simulink model "TBRe18_ECU_V7_AI"  (R2017b)
settings: Solver=FixedStepDiscrete  StartTime=0.0  StopTime=inf  FixedStep=0.0001  RelTol=1e-3
PostLoadFcn:
  | model_init();
libraries: simulink x16, simulink_extras x1
(part 1 of 4)
settings Model: SimulationMode=external  Creator=agf25  LastModifiedBy=kh469
settings DataIOCC: LimitDataPoints=on
settings OptimizationCC: DefaultParameterBehavior=Inlined  EfficientFloat2IntCast=on  LifeSpan=inf
settings DebuggingCC: AllowSymbolicDim=off  SFUnexpectedBacktrackingDiag=warning  SFNoUnconditionalDefaultTransitionDiag=warning  SFExecutionAtInitializationDiag=none
settings ModelReferenceCC: PropagateSignalLabelsOutOfModel=off
settings RTWCC: SystemTargetFile=nsi_mpc.tlc  MakeCommand=nsi_make  TemplateMakefile=nsi_mpc.tmf  Description=RTW Coder for MUXLAB4
settings CodeAppCC: StateflowObjectComments=on
settings STFCustomTargetCC: MATLABClassNameForMDSCustomization=Simulink.SoftwareTarget.TargetSpecificTriggerConfigurationBase  SystemTargetFile=nsi_mpc.tlc
settings ConfigComp: CovMetricSettings=dw  CovHtmlReporting=on  CovSaveCumulativeToWorkspaceVar=on  CovSaveSingleToWorkspaceVar=on  CovExternalEMLEnable=off
settings SimscapeCC: SimscapeNormalizeSystem=off
settings ConfigurationSet: Description=SimMechanics 2G

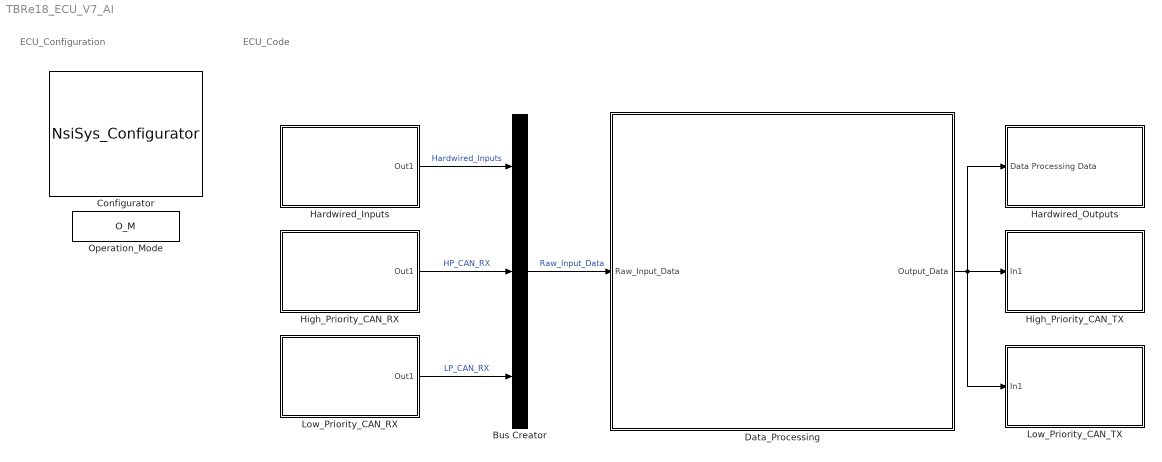
== system TBRe18_ECU_V7_AI ==
  note: ECU_Code
  note: ECU_Configuration
  Bus Creator : BusCreator  Inputs=3
  Configurator : S-Function  FunctionName=NsiSys_Configurator  Parameters=main,io,nbof_can,can,ccp,flash,nbof_lin,lin,tasks  SFunctionDeploymentMode=off  EnableBusSupport=off  mask(Configurator block){main=Config description;01/01/2011;0;0.000000, io=2.5;0;1;1;0;0;1;1;1, nbof_can=5, can=1;HIGH_SPEED;500Kbps;120 Ohm;C:\Users\TBRe-admin\Documents\MATLAB\TBRe18_DBC_190304.dbc;0;1;1Mbits;1;HIGH_SPEED;500Kbps;120 Ohm;C:\Users\TBRe-admin\Documents\MATLAB\TBRe18_DBC_190304.dbc;0;1;1Mbits;0;HIGH_SPEED;500Kbps;120 Ohm;C:\Users\l\Desktop\FYP\ECU\DBC\TBRe_DBC_V2.dbc;0;0;1Mbits;0;HIGH_SPEED;500Kbps;120 Ohm;D:\TOOLS\MUXLINK\R2011b\MUXlink\misc\j1939_adapt.dbc;0;1;1Mbits;0;HIGH_SPEED;1000Kbps;No;D:\TOOLS\MUXLINK\R2011b\MUXlink\misc\BASE_CAN_MUXLAB4.dbc;0;0;1Mbits, ccp=0;0x100;0x200;0;0;0x0;0x0;0;0x13, flash=Vehicle_STATE;No;Unsigned Byte;0;1;Operational_STATE;No;Unsigned Byte;0;1;Buzzer_time;No;Unsigned Byte;254;1;Buzzer_on;No;Boolean;1;1;reset_MEM;No;Boolean;0;1;TC_Slip_target;No;Unsigned Byte;5;1;TC_P_Gain;No;Unsigned Byte;1;1;TC_I_Gain;No;Unsigned Byte;1;1;TC_Offset;No;Signed Byte;0;1;DM_Mode;No;Unsigned Byte;0;1;DM_I_Gain;No;Unsigned Byte;1;1;IMD_MEM;No;Boolean;0;1;status_vehcle_LV;No;Boolean;0;1;status_vehcle_HV;No;Boolean;0;1;status_BMS;No;Boolean;0;1;status_IMD;No;Boolean;0;1;status_APPC;No;Boolean;0;1;status_APPS_BPPC;No;Boolean;0;1;status_RTD;No;Boolean;0;1;status_TC;No;Boolean;0;1;status_power_lim;No;Boolean;0;1;status_torque_derate;No;Boolean;0;1;status_tyre_radius;No;Unsigned Byte;22;1;power_limit;No;Unsigned Byte;30;1;torque_limit;No;Unsigned Byte;100;1, nbof_lin=2, lin=0;D:\TOOLS\MUXLINK\R2011b\MUXlink\misc\lindb.ldf;1;0.0;0.0;0.000;0.000;0.000000;0,0;0;D:\TOOLS\MUXLINK\R2011b\MUXlink\misc\lindb.ldf;1;0.0;0.0;0.000;0.000;0.000000;0,0, tasks=Data_Processing;[0.05];Hardwired_Inputs;[0.05];Hardwired_Outputs;[0.1];High_Priority_CAN_RX;[0.05];High_Priority_CAN_TX;[0.05];Low_Priority_CAN_RX;[0.05];Low_Priority_CAN_TX;[0.1]}
      mask prompts: nbof_can "nbof can"
      mask help: This block permits to set general parameters to use a MUXlink model
      mask init:
      | NsiSys_Configurator_InitializationFcn();
      settings: OpenFcn=NsiSys_Configurator_OpenFcn();
      mask Help:
      | eval('block=get_param(gcb, ''RTWdata'');')
      | web([docroot '\toolbox\MUXlink\html\blocks/' block.MUXlink_BlockType '.html'])
      mask Callback main: NsiSys_Configurator_ApplyFcn(1);
      mask Callback io: NsiSys_Configurator_ApplyFcn(2);
      mask Callback nbof_can: NsiSys_Configurator_ApplyFcn(3);
      mask Callback can: NsiSys_Configurator_ApplyFcn(4);
      mask Callback ccp: NsiSys_Configurator_ApplyFcn(5);
      mask Callback flash: NsiSys_Configurator_ApplyFcn(6);
      mask Callback nbof_lin: NsiSys_Configurator_ApplyFcn(7);
      mask Callback lin: NsiSys_Configurator_ApplyFcn(8);
      mask Callback tasks: NsiSys_Configurator_ApplyFcn(9);
      mask Display: image(imread('MUXLAB4.bmp'));text(0.5, 0.2, '', 'horizontalAlignment', 'center', 'verticalAlignment', 'base');
  Data_Processing : Subsystem  TreatAsAtomicUnit=on  SystemSampleTime=[0.05]  RTWFcnName=Data_Processing  RTWFileName=FileTaskFcn
      mask init:
      | NsiSys_SubSystemTask_InitializationFcn();
      settings: OpenFcn=NsiSys_SubSystemTask_OpenFcn();  RTWSystemCode=Nonreusable function  RTWFcnNameOpts=User specified  RTWFileNameOpts=Use function name
      mask Display: image(imread('nsi.bmp'));text(0.45, 0.9, 'task()');plot([0.05 0.05 0.05 0.05 0.05 0.05 0.05 0.05 0.05 0.05]);fprintf('Data_Processing\n/ 50.0ms / 10.0ms /\nEvent');
  Hardwired_Inputs : Subsystem  TreatAsAtomicUnit=on  SystemSampleTime=[0.05]  RTWFcnName=Hardwired_Inputs  RTWFileName=FileTaskFcn
      mask init:
      | NsiSys_SubSystemTask_InitializationFcn();
      settings: OpenFcn=NsiSys_SubSystemTask_OpenFcn();  RTWSystemCode=Nonreusable function  RTWFcnNameOpts=User specified  RTWFileNameOpts=Use function name
      mask Display: image(imread('nsi.bmp'));text(0.45, 0.9, 'task()');plot([0.05 0.05 0.05 0.05 0.05 0.05 0.05 0.05 0.05 0.05]);fprintf('Hardwired_Inputs\n/ 50.0ms / 0.0ms /\nEvent');
  Hardwired_Outputs : Subsystem  TreatAsAtomicUnit=on  SystemSampleTime=[0.1]  RTWFcnName=Hardwired_Outputs  RTWFileName=FileTaskFcn
      mask init:
      | NsiSys_SubSystemTask_InitializationFcn();
      settings: OpenFcn=NsiSys_SubSystemTask_OpenFcn();  RTWSystemCode=Nonreusable function  RTWFcnNameOpts=User specified  RTWFileNameOpts=Use function name
      mask Display: image(imread('nsi.bmp'));text(0.45, 0.9, 'task()');plot([0.05 0.05 0.05 0.05 0.05 0.05 0.05 0.05 0.05 0.05]);fprintf('Hardwired_Outputs\n/ 100.0ms / 0.0ms /\nEvent');
  High_Priority_CAN_RX : Subsystem  TreatAsAtomicUnit=on  SystemSampleTime=[0.05]  RTWFcnName=High_Priority_CAN_RX  RTWFileName=FileTaskFcn
      mask init:
      | NsiSys_SubSystemTask_InitializationFcn();
      settings: OpenFcn=NsiSys_SubSystemTask_OpenFcn();  RTWSystemCode=Nonreusable function  RTWFcnNameOpts=User specified  RTWFileNameOpts=Use function name
      mask Display: image(imread('nsi.bmp'));text(0.45, 0.9, 'task()');plot([0.05 0.05 0.05 0.05 0.05 0.05 0.05 0.05 0.05 0.05]);fprintf('High_Priority_CAN_RX\n/ 50.0ms / 0.0ms /\nEvent');
  High_Priority_CAN_TX : Subsystem  TreatAsAtomicUnit=on  SystemSampleTime=[0.05]  RTWFcnName=High_Priority_CAN_TX  RTWFileName=FileTaskFcn
      mask init:
      | NsiSys_SubSystemTask_InitializationFcn();
      settings: OpenFcn=NsiSys_SubSystemTask_OpenFcn();  RTWSystemCode=Nonreusable function  RTWFcnNameOpts=User specified  RTWFileNameOpts=Use function name
      mask Display: image(imread('nsi.bmp'));text(0.45, 0.9, 'task()');plot([0.05 0.05 0.05 0.05 0.05 0.05 0.05 0.05 0.05 0.05]);fprintf('High_Priority_CAN_TX\n/ 50.0ms / 20.0ms /\nEvent');
  Low_Priority_CAN_RX : Subsystem  TreatAsAtomicUnit=on  SystemSampleTime=[0.05]  RTWFcnName=Low_Priority_CAN_RX  RTWFileName=FileTaskFcn
      mask init:
      | NsiSys_SubSystemTask_InitializationFcn();
      settings: OpenFcn=NsiSys_SubSystemTask_OpenFcn();  RTWSystemCode=Nonreusable function  RTWFcnNameOpts=User specified  RTWFileNameOpts=Use function name
      mask Display: image(imread('nsi.bmp'));text(0.45, 0.9, 'task()');plot([0.05 0.05 0.05 0.05 0.05 0.05 0.05 0.05 0.05 0.05]);fprintf('Low_Priority_CAN_RX\n/ 50.0ms / 0.0ms /\nEvent');
  Low_Priority_CAN_TX : Subsystem  TreatAsAtomicUnit=on  SystemSampleTime=[0.1]  RTWFcnName=Low_Priority_CAN_TX  RTWFileName=FileTaskFcn
      mask init:
      | NsiSys_SubSystemTask_InitializationFcn();
      settings: OpenFcn=NsiSys_SubSystemTask_OpenFcn();  RTWSystemCode=Nonreusable function  RTWFcnNameOpts=User specified  RTWFileNameOpts=Use function name
      mask Display: image(imread('nsi.bmp'));text(0.45, 0.9, 'task()');plot([0.05 0.05 0.05 0.05 0.05 0.05 0.05 0.05 0.05 0.05]);fprintf('Low_Priority_CAN_TX\n/ 100.0ms / 0.0ms /\nEvent');
  Operation_Mode : DataStoreMemory  DataStoreName=O_M  ReadBeforeWriteMsg=warning  WriteAfterWriteMsg=warning  WriteAfterReadMsg=warning  ShowAdditionalParam=off
  wires:
  Low_Priority_CAN_RX/1(Out1) -> Bus Creator/3  "LP_CAN_RX"
  High_Priority_CAN_RX/1(Out1) -> Bus Creator/2  "HP_CAN_RX"
  Hardwired_Inputs/1(Out1) -> Bus Creator/1  "Hardwired_Inputs"
  Bus Creator/1 -> Data_Processing/1(Raw_Input_Data)  "Raw_Input_Data"
  Data_Processing/1(Output_Data) -> Low_Priority_CAN_TX/1(In1), High_Priority_CAN_TX/1(In1), Hardwired_Outputs/1(Data Processing Data)

== system TBRe18_ECU_V7_AI/Data_Processing ==
  note: Data_Processing
  Raw_Input_Data : Inport
  Diagnostics : Subsystem
  Init : Subsystem  mask(System Initialize){}
      mask help: Add code to a systems Initialize function
      settings: CopyFcn=cccopyfcn(gcb)  OpenFcn=ccopenfcn('System Initialize Function')
      mask Help: This block contains text fields to insert custom user code sections at the declaration, execution and exit sections of the systems initialize function.  By placing this block inside a subsytem, the custom user code will appear in that subsystems function.
      mask Display: disp('I()')
  Signal Conversion : SignalConversion  OverrideOpt=off
  Task : S-Function  FunctionName=NsiSys_TaskREF  Parameters=task_initialised,task_periodic, task_sampletime,task_name,task_event,task_offset  SFunctionDeploymentMode=off  EnableBusSupport=off  mask(task definition){task_initialised=on, task_periodic=on, task_sampletime=[0.05], task_offset=0.01, task_name=Data_Processing, task_event=on}
      mask prompts: task_initialised "task initialised"; task_periodic "Is Periodic"; task_sampletime "Task sample time"; task_offset "Task Offset"; task_name "Task name"; task_event "Is event"
      mask help:
      | Permit to provide all parameters associated to a MUXLINK task.
      | Task can be executed periodicaly and/or on event detection.
      | If task is periodic:
      | Task sample time specify the execution period in mS [0.001   6000]
      | Task Offset specify the offset applied to the execution period
      | Task Offset < Task sample time
      mask init:
      | NsiSys_TaskREF_InitializationFcn();
      settings: OpenFcn=NsiSys_Task_OpenFcn();
      mask Callback task_initialised: NsiSys_TaskREF_ApplyFcn(1);
      mask Callback task_periodic: NsiSys_TaskREF_ApplyFcn(2);
      mask Callback task_sampletime: NsiSys_TaskREF_ApplyFcn(3);
      mask Callback task_offset: NsiSys_TaskREF_ApplyFcn(6);
      mask Callback task_name: NsiSys_TaskREF_ApplyFcn(4);
      mask Callback task_event: NsiSys_TaskREF_ApplyFcn(5);
      mask Display: text(0.5, 0.8, 't()', 'horizontalAlignment', 'center', 'verticalAlignment', 'base');text(0.5, 0.2, '/ 50.0ms / 10.0ms /', 'horizontalAlignment', 'center', 'verticalAlignment', 'base');text(0.5, 0.4, 'Event', 'horizontalAlignment', 'center', 'verticalAlignment', 'base');
  Vehicle_Functionality : Subsystem
  Output_Data : Outport
  wires:
  Raw_Input_Data/1 -> Signal Conversion/1
  Diagnostics/1(Input_Data_Bus) -> Vehicle_Functionality/1(Input_Data)
  Signal Conversion/1 -> Diagnostics/1(Raw_Input_Data)
  Vehicle_Functionality/1(Output_Data_Bus) -> Output_Data/1

== system TBRe18_ECU_V7_AI/Hardwired_Inputs ==
  AnalogInput2 : S-Function  FunctionName=NsiIo_AnalogInput  Parameters=channel  SFunctionDeploymentMode=off  EnableBusSupport=off  mask(MUXlink I/O Analog Input){channel=7, RANGE=0 / 20 Volts}
      mask prompts: channel "Channel ?"; RANGE "Plage de mesure"
      mask help: This block interface the 8 Analog Inputs. Channels 1 to 4 are 0/10V, and the channels 5 to 8 are0/20V. Voltage input is read in mV
      mask init:
      | NsiIo_AnalogInput_InitializationFcn();
      settings: OpenFcn=NsiIo_AnalogInput_OpenFcn();
      mask Help:
      | eval('block=get_param(gcb, ''RTWdata'');')
      | web([docroot '\toolbox\MUXlink\html\blocks/' block.MUXlink_BlockType '.html'])
      mask Callback channel: NsiIo_AnalogInput_ApplyFcn();
      mask Callback RANGE: NsiIo_AnalogInput_ApplyFcn();
      mask Display: image(imread('nsi.bmp'));text(0.5, 0.2, 'AnalogInput_7\n\n0 / 20 Volts', 'horizontalAlignment', 'center', 'verticalAlignment', 'base');plot([0.05 0.05 0.05 0.05 0.05 0.05 0.05 0.05 0.05 0.05]);port_label('output', 1, 'D3');
  Bus Creator : BusCreator  Inputs=7
  Console : Subsystem
  DigitalInput1 : S-Function  FunctionName=NsiIo_DigitalInput  Parameters=channel,is_trigger,typeof_trigger,is_wakeup,wakeup_level  SFunctionDeploymentMode=off  EnableBusSupport=off  mask(MUXlink I/O Digital Input){channel=6, is_trigger=off, typeof_trigger=Either, is_wakeup=off, wakeup_level=Low level}
      mask prompts: channel "Channel ?"; is_trigger "Trigger ?"; typeof_trigger "Type of Trigger ?"; is_wakeup "Wake-up ?"; wakeup_level "Wake-up level ?"
      mask help: Read digital input from I/O channel.
      mask init:
      | NsiIo_DigitalInput_InitializationFcn();
      settings: OpenFcn=NsiIo_DigitalInput_OpenFcn();
      mask Help:
      | eval('block=get_param(gcb, ''RTWdata'');')
      | web([docroot '\toolbox\MUXlink\html\blocks/' block.MUXlink_BlockType '.html'])
      mask Callback channel: NsiIo_DigitalInput_ApplyFcn(1);
      mask Callback is_trigger: NsiIo_DigitalInput_ApplyFcn(2);
      mask TypeOptions typeof_trigger: Rising | Falling | Either
      mask Callback typeof_trigger: NsiIo_DigitalInput_ApplyFcn(3);
      mask Callback is_wakeup: NsiIo_DigitalInput_ApplyFcn(4);
      mask TypeOptions wakeup_level: Low level | High level
      mask Callback wakeup_level: NsiIo_DigitalInput_ApplyFcn(5);
      mask Display: image(imread('nsi.bmp'));text(0.5, 0.2, 'DigitalInput_6', 'horizontalAlignment', 'center', 'verticalAlignment', 'base');plot([0.05 0.05 0.05 0.05 0.05 0.05 0.05 0.05 0.05 0.05]);port_label('output', 1, 'Ground : B2');
  Ground : Ground
  Ground1 : Ground
  Init : Subsystem  mask(System Initialize){}
      mask help: Add code to a systems Initialize function
      settings: CopyFcn=cccopyfcn(gcb)  OpenFcn=ccopenfcn('System Initialize Function')
      mask Help: This block contains text fields to insert custom user code sections at the declaration, execution and exit sections of the systems initialize function.  By placing this block inside a subsytem, the custom user code will appear in that subsystems function.
      mask Display: disp('I()')
  Pedal_Box : Subsystem
  Task : S-Function  FunctionName=NsiSys_TaskREF  Parameters=task_initialised,task_periodic, task_sampletime,task_name,task_event,task_offset  SFunctionDeploymentMode=off  EnableBusSupport=off  mask(task definition){task_initialised=on, task_periodic=on, task_sampletime=[0.05], task_offset=0.0, task_name=Hardwired_Inputs, task_event=on}
      mask prompts: task_initialised "task initialised"; task_periodic "Is Periodic"; task_sampletime "Task sample time"; task_offset "Task Offset"; task_name "Task name"; task_event "Is event"
      mask help:
      | Permit to provide all parameters associated to a MUXLINK task.
      | Task can be executed periodicaly and/or on event detection.
      | If task is periodic:
      | Task sample time specify the execution period in mS [0.001   6000]
      | Task Offset specify the offset applied to the execution period
      | Task Offset < Task sample time
      mask init:
      | NsiSys_TaskREF_InitializationFcn();
      settings: OpenFcn=NsiSys_Task_OpenFcn();
      mask Callback task_initialised: NsiSys_TaskREF_ApplyFcn(1);
      mask Callback task_periodic: NsiSys_TaskREF_ApplyFcn(2);
      mask Callback task_sampletime: NsiSys_TaskREF_ApplyFcn(3);
      mask Callback task_offset: NsiSys_TaskREF_ApplyFcn(6);
      mask Callback task_name: NsiSys_TaskREF_ApplyFcn(4);
      mask Callback task_event: NsiSys_TaskREF_ApplyFcn(5);
      mask Display: text(0.5, 0.8, 't()', 'horizontalAlignment', 'center', 'verticalAlignment', 'base');text(0.5, 0.2, '/ 50.0ms / 0.0ms /', 'horizontalAlignment', 'center', 'verticalAlignment', 'base');text(0.5, 0.4, 'Event', 'horizontalAlignment', 'center', 'verticalAlignment', 'base');
  VBat : S-Function  FunctionName=NsiIo_Vbat  SFunctionDeploymentMode=off  EnableBusSupport=off  mask(MUXlink I/O VBat){}
      mask help: Battery Voltage
      mask init:
      | NsiIo_Vbat_InitializationFcn();
      settings: OpenFcn=NsiIo_Vbat_OpenFcn();
      mask Help:
      | eval('block=get_param(gcb, ''RTWdata'');')
      | web([docroot '\toolbox\MUXlink\html\blocks/' block.MUXlink_BlockType '.html'])
      mask Display: image(imread('nsi.bmp'));text(0.5, 0.2, 'I/O VBat', 'horizontalAlignment', 'center', 'verticalAlignment', 'base');plot([0.05 0.05 0.05 0.05 0.05 0.05 0.05 0.05 0.05 0.05]);port_label('output', 1, 'Voltage');
  Out1 : Outport
  wires:
  Pedal_Box/1(Out1) -> Bus Creator/1  "Pedal_Box_Data"
  Console/1(Out1) -> Bus Creator/2  "Console_Data"
  Bus Creator/1 -> Out1/1
  VBat/1 -> Bus Creator/3  "LV_Battery_Voltage"
  AnalogInput2/1 -> Bus Creator/7  "AMS_Ok"
  Ground/1 -> Bus Creator/4
  Ground1/1 -> Bus Creator/6
  DigitalInput1/1 -> Bus Creator/5  "RTD_Driverless"

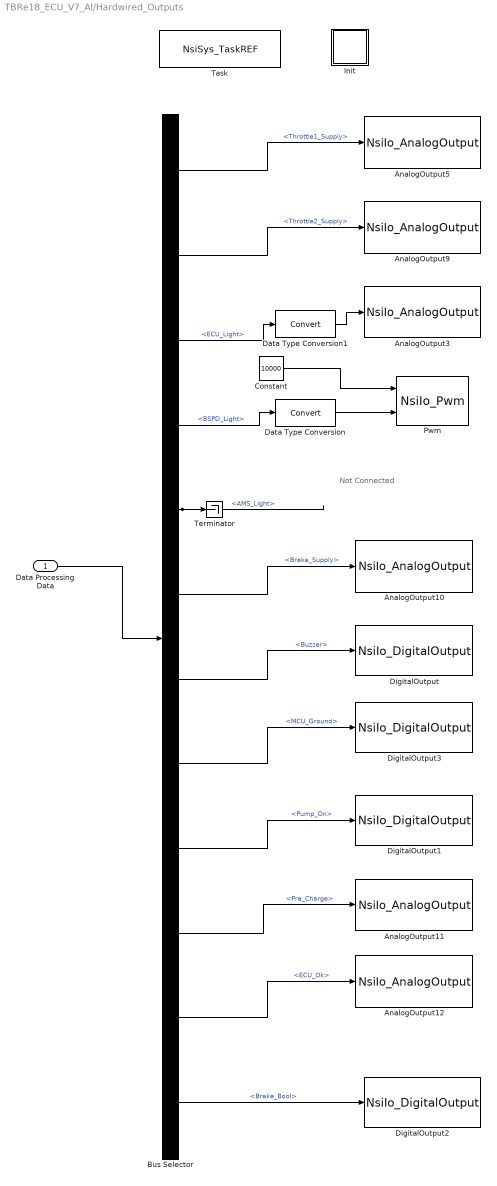
== system TBRe18_ECU_V7_AI/Hardwired_Outputs ==
  note: Not Connected
  Data Processing Data : Inport
  AnalogOutput10 : S-Function  Description=fsgqsdgqsgqsqs\nqdsjfhkqfkqsd  FunctionName=NsiIo_AnalogOutput  Parameters=Channel,Feedback  SFunctionDeploymentMode=off  EnableBusSupport=off  mask(MUXlink I/O Analog Output){Channel=5, Feedback=off, RANGE=0 / 20 Volts}
      mask prompts: Channel "Channel ?"; Feedback "Read Back Analog out"; RANGE "Voltage Range"
      mask help: This block interface the 8 Analog Outputs. Channels 1 to 4 are 0/10V, and the channels 5 to 8 are0/20V. Voltage input is set in mV
      mask init:
      | NsiIo_AnalogOutput_InitializationFcn();
      settings: OpenFcn=NsiIo_AnalogOutput_OpenFcn();
      mask Help:
      | eval('block=get_param(gcb, ''RTWdata'');')
      | web([docroot '\toolbox\MUXlink\html\blocks/' block.MUXlink_BlockType '.html'])
      mask Callback Channel: NsiIo_AnalogOutput_ApplyFcn(1);
      mask Display: image(imread('nsi.bmp'));text(0.5, 0.2, 'AnalogOutput_5\n\n0 / 20 Volts', 'horizontalAlignment', 'center', 'verticalAlignment', 'base');plot([0.05 0.05 0.05 0.05 0.05 0.05 0.05 0.05 0.05 0.05]);port_label('input', 1, 'F3');
  AnalogOutput11 : S-Function  Description=fsgqsdgqsgqsqs\nqdsjfhkqfkqsd  FunctionName=NsiIo_AnalogOutput  Parameters=Channel,Feedback  SFunctionDeploymentMode=off  EnableBusSupport=off  mask(MUXlink I/O Analog Output){Channel=7, Feedback=off, RANGE=0 / 20 Volts}
      mask prompts: Channel "Channel ?"; Feedback "Read Back Analog out"; RANGE "Voltage Range"
      mask help: This block interface the 8 Analog Outputs. Channels 1 to 4 are 0/10V, and the channels 5 to 8 are0/20V. Voltage input is set in mV
      mask init:
      | NsiIo_AnalogOutput_InitializationFcn();
      settings: OpenFcn=NsiIo_AnalogOutput_OpenFcn();
      mask Help:
      | eval('block=get_param(gcb, ''RTWdata'');')
      | web([docroot '\toolbox\MUXlink\html\blocks/' block.MUXlink_BlockType '.html'])
      mask Callback Channel: NsiIo_AnalogOutput_ApplyFcn(1);
      mask Display: image(imread('nsi.bmp'));text(0.5, 0.2, 'AnalogOutput_7\n\n0 / 20 Volts', 'horizontalAlignment', 'center', 'verticalAlignment', 'base');plot([0.05 0.05 0.05 0.05 0.05 0.05 0.05 0.05 0.05 0.05]);port_label('input', 1, 'A2');
  AnalogOutput12 : S-Function  Description=fsgqsdgqsgqsqs\nqdsjfhkqfkqsd  FunctionName=NsiIo_AnalogOutput  Parameters=Channel,Feedback  SFunctionDeploymentMode=off  EnableBusSupport=off  mask(MUXlink I/O Analog Output){Channel=2, Feedback=off, RANGE=0 / 20 Volts}
      mask prompts: Channel "Channel ?"; Feedback "Read Back Analog out"; RANGE "Voltage Range"
      mask help: This block interface the 8 Analog Outputs. Channels 1 to 4 are 0/10V, and the channels 5 to 8 are0/20V. Voltage input is set in mV
      mask init:
      | NsiIo_AnalogOutput_InitializationFcn();
      settings: OpenFcn=NsiIo_AnalogOutput_OpenFcn();
      mask Help:
      | eval('block=get_param(gcb, ''RTWdata'');')
      | web([docroot '\toolbox\MUXlink\html\blocks/' block.MUXlink_BlockType '.html'])
      mask Callback Channel: NsiIo_AnalogOutput_ApplyFcn(1);
      mask Display: image(imread('nsi.bmp'));text(0.5, 0.2, 'AnalogOutput_2\n\n0 / 20 Volts', 'horizontalAlignment', 'center', 'verticalAlignment', 'base');plot([0.05 0.05 0.05 0.05 0.05 0.05 0.05 0.05 0.05 0.05]);port_label('input', 1, 'E4');
  AnalogOutput3 : S-Function  Description=fsgqsdgqsgqsqs\nqdsjfhkqfkqsd  FunctionName=NsiIo_AnalogOutput  Parameters=Channel,Feedback  SFunctionDeploymentMode=off  EnableBusSupport=off  mask(MUXlink I/O Analog Output){Channel=6, Feedback=off, RANGE=0 / 20 Volts}
      mask prompts: Channel "Channel ?"; Feedback "Read Back Analog out"; RANGE "Voltage Range"
      mask help: This block interface the 8 Analog Outputs. Channels 1 to 4 are 0/10V, and the channels 5 to 8 are0/20V. Voltage input is set in mV
      mask init:
      | NsiIo_AnalogOutput_InitializationFcn();
      settings: OpenFcn=NsiIo_AnalogOutput_OpenFcn();
      mask Help:
      | eval('block=get_param(gcb, ''RTWdata'');')
      | web([docroot '\toolbox\MUXlink\html\blocks/' block.MUXlink_BlockType '.html'])
      mask Callback Channel: NsiIo_AnalogOutput_ApplyFcn(1);
      mask Display: image(imread('nsi.bmp'));text(0.5, 0.2, 'AnalogOutput_6\n\n0 / 20 Volts', 'horizontalAlignment', 'center', 'verticalAlignment', 'base');plot([0.05 0.05 0.05 0.05 0.05 0.05 0.05 0.05 0.05 0.05]);port_label('input', 1, 'F4');
  AnalogOutput5 : S-Function  Description=fsgqsdgqsgqsqs\nqdsjfhkqfkqsd  FunctionName=NsiIo_AnalogOutput  Parameters=Channel,Feedback  SFunctionDeploymentMode=off  EnableBusSupport=off  mask(MUXlink I/O Analog Output){Channel=3, Feedback=off, RANGE=0 / 20 Volts}
      mask prompts: Channel "Channel ?"; Feedback "Read Back Analog out"; RANGE "Voltage Range"
      mask help: This block interface the 8 Analog Outputs. Channels 1 to 4 are 0/10V, and the channels 5 to 8 are0/20V. Voltage input is set in mV
      mask init:
      | NsiIo_AnalogOutput_InitializationFcn();
      settings: OpenFcn=NsiIo_AnalogOutput_OpenFcn();
      mask Help:
      | eval('block=get_param(gcb, ''RTWdata'');')
      | web([docroot '\toolbox\MUXlink\html\blocks/' block.MUXlink_BlockType '.html'])
      mask Callback Channel: NsiIo_AnalogOutput_ApplyFcn(1);
      mask Display: image(imread('nsi.bmp'));text(0.5, 0.2, 'AnalogOutput_3\n\n0 / 20 Volts', 'horizontalAlignment', 'center', 'verticalAlignment', 'base');plot([0.05 0.05 0.05 0.05 0.05 0.05 0.05 0.05 0.05 0.05]);port_label('input', 1, 'F1');
  AnalogOutput9 : S-Function  Description=fsgqsdgqsgqsqs\nqdsjfhkqfkqsd  FunctionName=NsiIo_AnalogOutput  Parameters=Channel,Feedback  SFunctionDeploymentMode=off  EnableBusSupport=off  mask(MUXlink I/O Analog Output){Channel=4, Feedback=off, RANGE=0 / 20 Volts}
      mask prompts: Channel "Channel ?"; Feedback "Read Back Analog out"; RANGE "Voltage Range"
      mask help: This block interface the 8 Analog Outputs. Channels 1 to 4 are 0/10V, and the channels 5 to 8 are0/20V. Voltage input is set in mV
      mask init:
      | NsiIo_AnalogOutput_InitializationFcn();
      settings: OpenFcn=NsiIo_AnalogOutput_OpenFcn();
      mask Help:
      | eval('block=get_param(gcb, ''RTWdata'');')
      | web([docroot '\toolbox\MUXlink\html\blocks/' block.MUXlink_BlockType '.html'])
      mask Callback Channel: NsiIo_AnalogOutput_ApplyFcn(1);
      mask Display: image(imread('nsi.bmp'));text(0.5, 0.2, 'AnalogOutput_4\n\n0 / 20 Volts', 'horizontalAlignment', 'center', 'verticalAlignment', 'base');plot([0.05 0.05 0.05 0.05 0.05 0.05 0.05 0.05 0.05 0.05]);port_label('input', 1, 'F2');
  Bus Selector : BusSelector  OutputSignals=Hardwired_Output_Data.Throttle1_Supply,Hardwired_Output_Data.Throttle2_Supply,Hardwired_Output_Data.ECU_Light,Hardwired_Output_Data.BSPD_Light,Hardwired_Output_Data.AMS_Light,Hardwired_Output_Data.Brake_Supply,Vehicle_Operation_Data.Buzzer,Hardwired_Output_Data.MCU_Ground,Hardwired_Output_Data.Pump_On,Hardwired_Output_Data.Pre_Charge,Hardwired_Output_Data.ECU_Ok,Vehicle_Operation_Data.Brake_Bool
  Constant : Constant  Value=10000  OutDataTypeStr=uint32
  Data Type Conversion : DataTypeConversion
  Data Type Conversion1 : DataTypeConversion
  DigitalOutput : S-Function  FunctionName=NsiIo_DigitalOutput  Parameters=channel,side,feedback  SFunctionDeploymentMode=off  EnableBusSupport=off  mask(MUXlink I/O Digital Output){channel=3, side=High, feedback=off}
      mask prompts: channel "Channel ?"; side "Side ?"; feedback "With feedback ?"
      mask help: Write Digital Output onto I/O channel.
      mask init:
      | NsiIo_DigitalOutput_InitializationFcn();
      settings: OpenFcn=NsiIo_DigitalOutput_OpenFcn();
      mask Help:
      | eval('block=get_param(gcb, ''RTWdata'');')
      | web([docroot '\toolbox\MUXlink\html\blocks/' block.MUXlink_BlockType '.html'])
      mask Callback channel: NsiIo_DigitalOutput_ApplyFcn(1);
      mask TypeOptions side: High | Low
      mask Callback side: NsiIo_DigitalOutput_ApplyFcn(2);
      mask Callback feedback: NsiIo_DigitalOutput_ApplyFcn(3);
      mask Display: image(imread('nsi.bmp'));text(0.5, 0.2, 'DigitalOutput_3', 'horizontalAlignment', 'center', 'verticalAlignment', 'base');plot([0.05 0.05 0.05 0.05 0.05 0.05 0.05 0.05 0.05 0.05]);port_label('input', 1, 'L3 : High Side');
  DigitalOutput1 : S-Function  FunctionName=NsiIo_DigitalOutput  Parameters=channel,side,feedback  SFunctionDeploymentMode=off  EnableBusSupport=off  mask(MUXlink I/O Digital Output){channel=1, side=High, feedback=off}
      mask prompts: channel "Channel ?"; side "Side ?"; feedback "With feedback ?"
      mask help: Write Digital Output onto I/O channel.
      mask init:
      | NsiIo_DigitalOutput_InitializationFcn();
      settings: OpenFcn=NsiIo_DigitalOutput_OpenFcn();
      mask Help:
      | eval('block=get_param(gcb, ''RTWdata'');')
      | web([docroot '\toolbox\MUXlink\html\blocks/' block.MUXlink_BlockType '.html'])
      mask Callback channel: NsiIo_DigitalOutput_ApplyFcn(1);
      mask TypeOptions side: High | Low
      mask Callback side: NsiIo_DigitalOutput_ApplyFcn(2);
      mask Callback feedback: NsiIo_DigitalOutput_ApplyFcn(3);
      mask Display: image(imread('nsi.bmp'));text(0.5, 0.2, 'DigitalOutput_1', 'horizontalAlignment', 'center', 'verticalAlignment', 'base');plot([0.05 0.05 0.05 0.05 0.05 0.05 0.05 0.05 0.05 0.05]);port_label('input', 1, 'G2 : High Side');
  DigitalOutput2 : S-Function  FunctionName=NsiIo_DigitalOutput  Parameters=channel,side,feedback  SFunctionDeploymentMode=off  EnableBusSupport=off  mask(MUXlink I/O Digital Output){channel=2, side=High, feedback=off}
      mask prompts: channel "Channel ?"; side "Side ?"; feedback "With feedback ?"
      mask help: Write Digital Output onto I/O channel.
      mask init:
      | NsiIo_DigitalOutput_InitializationFcn();
      settings: OpenFcn=NsiIo_DigitalOutput_OpenFcn();
      mask Help:
      | eval('block=get_param(gcb, ''RTWdata'');')
      | web([docroot '\toolbox\MUXlink\html\blocks/' block.MUXlink_BlockType '.html'])
      mask Callback channel: NsiIo_DigitalOutput_ApplyFcn(1);
      mask TypeOptions side: High | Low
      mask Callback side: NsiIo_DigitalOutput_ApplyFcn(2);
      mask Callback feedback: NsiIo_DigitalOutput_ApplyFcn(3);
      mask Display: image(imread('nsi.bmp'));text(0.5, 0.2, 'DigitalOutput_2', 'horizontalAlignment', 'center', 'verticalAlignment', 'base');plot([0.05 0.05 0.05 0.05 0.05 0.05 0.05 0.05 0.05 0.05]);port_label('input', 1, 'G3 : High Side');
  DigitalOutput3 : S-Function  FunctionName=NsiIo_DigitalOutput  Parameters=channel,side,feedback  SFunctionDeploymentMode=off  EnableBusSupport=off  mask(MUXlink I/O Digital Output){channel=1, side=Low, feedback=off}
      mask prompts: channel "Channel ?"; side "Side ?"; feedback "With feedback ?"
      mask help: Write Digital Output onto I/O channel.
      mask init:
      | NsiIo_DigitalOutput_InitializationFcn();
      settings: OpenFcn=NsiIo_DigitalOutput_OpenFcn();
      mask Help:
      | eval('block=get_param(gcb, ''RTWdata'');')
      | web([docroot '\toolbox\MUXlink\html\blocks/' block.MUXlink_BlockType '.html'])
      mask Callback channel: NsiIo_DigitalOutput_ApplyFcn(1);
      mask TypeOptions side: High | Low
      mask Callback side: NsiIo_DigitalOutput_ApplyFcn(2);
      mask Callback feedback: NsiIo_DigitalOutput_ApplyFcn(3);
      mask Display: image(imread('nsi.bmp'));text(0.5, 0.2, 'DigitalOutput_1', 'horizontalAlignment', 'center', 'verticalAlignment', 'base');plot([0.05 0.05 0.05 0.05 0.05 0.05 0.05 0.05 0.05 0.05]);port_label('input', 1, 'H2 : Low Side');
  Init : Subsystem  mask(System Initialize){}
      mask help: Add code to a systems Initialize function
      settings: CopyFcn=cccopyfcn(gcb)  OpenFcn=ccopenfcn('System Initialize Function')
      mask Help: This block contains text fields to insert custom user code sections at the declaration, execution and exit sections of the systems initialize function.  By placing this block inside a subsytem, the custom user code will appear in that subsystems function.
      mask Display: disp('I()')
  Pwm : S-Function  FunctionName=NsiIo_Pwm  Parameters=channel  SFunctionDeploymentMode=off  EnableBusSupport=off  mask(MUXlink I/O Pwm){channel=3}
      mask prompts: channel "Channel ?"
      mask help: Write value onto I/O PWM channel.
      mask init:
      | NsiIo_Pwm_InitializationFcn();
      settings: OpenFcn=NsiIo_Pwm_OpenFcn();
      mask Help:
      | eval('block=get_param(gcb, ''RTWdata'');')
      | web([docroot '\toolbox\MUXlink\html\blocks/' block.MUXlink_BlockType '.html'])
      mask Callback channel: NsiIo_Pwm_ApplyFcn(1);
      mask Display: image(imread('nsi.bmp'));text(0.5, 0.2, 'Pwm_3', 'horizontalAlignment', 'center', 'verticalAlignment', 'base');plot([0.05 0.05 0.05 0.05 0.05 0.05 0.05 0.05 0.05 0.05]);port_label('input', 1, 'Hz');port_label('input', 2, '%');text(0.1, 0.5, 'A1', 'horizontalAlignment','center');
  Task : S-Function  FunctionName=NsiSys_TaskREF  Parameters=task_initialised,task_periodic, task_sampletime,task_name,task_event,task_offset  SFunctionDeploymentMode=off  EnableBusSupport=off  mask(task definition){task_initialised=on, task_periodic=on, task_sampletime=[0.1], task_offset=0, task_name=Hardwired_Outputs, task_event=on}
      mask prompts: task_initialised "task initialised"; task_periodic "Is Periodic"; task_sampletime "Task sample time"; task_offset "Task Offset"; task_name "Task name"; task_event "Is event"
      mask help:
      | Permit to provide all parameters associated to a MUXLINK task.
      | Task can be executed periodicaly and/or on event detection.
      | If task is periodic:
      | Task sample time specify the execution period in mS [0.001   6000]
      | Task Offset specify the offset applied to the execution period
      | Task Offset < Task sample time
      mask init:
      | NsiSys_TaskREF_InitializationFcn();
      settings: OpenFcn=NsiSys_Task_OpenFcn();
      mask Callback task_initialised: NsiSys_TaskREF_ApplyFcn(1);
      mask Callback task_periodic: NsiSys_TaskREF_ApplyFcn(2);
      mask Callback task_sampletime: NsiSys_TaskREF_ApplyFcn(3);
      mask Callback task_offset: NsiSys_TaskREF_ApplyFcn(6);
      mask Callback task_name: NsiSys_TaskREF_ApplyFcn(4);
      mask Callback task_event: NsiSys_TaskREF_ApplyFcn(5);
      mask Display: text(0.5, 0.8, 't()', 'horizontalAlignment', 'center', 'verticalAlignment', 'base');text(0.5, 0.2, '/ 100.0ms / 0.0ms /', 'horizontalAlignment', 'center', 'verticalAlignment', 'base');text(0.5, 0.4, 'Event', 'horizontalAlignment', 'center', 'verticalAlignment', 'base');
  Terminator : Terminator
  wires:
  Data Processing Data/1 -> Bus Selector/1
  Bus Selector/1 -> AnalogOutput5/1  "<Throttle1_Supply>"
  Bus Selector/2 -> AnalogOutput9/1  "<Throttle2_Supply>"
  Bus Selector/7 -> DigitalOutput/1  "<Buzzer>"
  Bus Selector/9 -> DigitalOutput1/1  "<Pump_On>"
  Bus Selector/5 -> Terminator/1  "<AMS_Light>"
  Bus Selector/3 -> Data Type Conversion1/1  "<ECU_Light>"
  Bus Selector/11 -> AnalogOutput12/1  "<ECU_Ok>"
  Bus Selector/10 -> AnalogOutput11/1  "<Pre_Charge>"
  Bus Selector/6 -> AnalogOutput10/1  "<Brake_Supply>"
  Constant/1 -> Pwm/1
  Bus Selector/4 -> Data Type Conversion/1  "<BSPD_Light>"
  Bus Selector/12 -> DigitalOutput2/1  "<Brake_Bool>"
  Bus Selector/8 -> DigitalOutput3/1  "<MCU_Ground>"
  Data Type Conversion/1 -> Pwm/2
  Data Type Conversion1/1 -> AnalogOutput3/1

== system TBRe18_ECU_V7_AI/High_Priority_CAN_RX ==
  Bus Creator1 : BusCreator  Inputs=9
  CanRx2 : S-Function  FunctionName=NsiCan_Rx_Ext  Parameters=data_can,channel,msg_name,ident,ident_type,dlc,signals,is_trigger,is_physical,is_canfd,is_rxgw  SFunctionDeploymentMode=off  EnableBusSupport=off  mask(MUXlink Can Rx){data_can=1;HIGH_SPEED;500Kbps;120 Ohm;C:\Users\TBRe-admin\Documents\MATLAB\TBRe18_DBC_190304.dbc;0;;;1;LOW_SPEED;125Kbps;560 Ohm;C:\Users\TBRe-admin\Documents\MATLAB\TBRe18_DBC_190304.dbc;0;;;0;HIGH_SPEED;1000Kbps;120 Ohm;D:\TOOLS\MUXLINK\R2011b\MUXlink\misc\BASE_CAN_MUXLAB4.dbc;0;;;0;HIGH_SPEED;500Kbps;120 Ohm;D:\TOOLS\MUXLINK\R2011b\MUXlink\misc\j1939_adapt.dbc;0;;;0;HIGH_SPEED;1000Kbps;No;D:\TOOLS\MUXLINK\R2011b\MUXlink\misc\BASE_CAN_MUXLAB4.dbc;0;;, channel=1, msg_name=MCU_TPDO2, ident=0x281, ident_type=STD, dlc=8, signals=Motor_Temp;1;8;8;1.000000;0.000000;_;MCU_Temp;1;0;8;1.000000;0.000000;_;MCU_DC_Link_Voltage;1;16;-16;1.000000;0.000000;_;MCU_DC_Link_Current;1;32;-32;1.000000;0.000000;_, is_trigger=0, is_physical=0, is_canfd=0, is_rxgw=0}
      mask prompts: data_can "data can"; msg_name "msg name"
      mask help: Receive a frame from a CAN channel.
      mask init:
      | NsiCan_Rx_Ext_InitializationFcn();
      settings: OpenFcn=NsiCan_Rx_Ext_OpenFcn();
      mask Help:
      | eval('block=get_param(gcb, ''RTWdata'');')
      | web([docroot '\toolbox\MUXlink\html\blocks/' block.MUXlink_BlockType '.html'])
      mask Callback data_can: NsiCan_Rx_Ext_ApplyFcn(1);
      mask Callback channel: NsiCan_Rx_Ext_ApplyFcn(2);
      mask Callback msg_name: NsiCan_Rx_Ext_ApplyFcn(3);
      mask Callback ident: NsiCan_Rx_Ext_ApplyFcn(4);
      mask Callback ident_type: NsiCan_Rx_Ext_ApplyFcn(5);
      mask Callback dlc: NsiCan_Rx_Ext_ApplyFcn(6);
      mask Callback signals: NsiCan_Rx_Ext_ApplyFcn(7);
      mask Callback is_trigger: NsiCan_Rx_Ext_ApplyFcn(8);
      mask Callback is_physical: NsiCan_Rx_Ext_ApplyFcn(9);
      mask Callback is_canfd: NsiCan_Rx_Ext_ApplyFcn(10);
      mask Callback is_rxgw: NsiCan_Rx_Ext_ApplyFcn(11);
      mask Display: image(imread('nsi.bmp'));text(0.5, 0.3, 'RX_MCU_TPDO2_CAN1', 'horizontalAlignment', 'center', 'verticalAlignment', 'base');plot([0.05 0.05 0.05 0.05 0.05 0.05 0.05 0.05 0.05 0.05]); port_label('output',1, 'Motor_Temp'); port_label('output',2, 'MCU_Temp'); port_label('output',3, 'MCU_DC_Link_Voltage'); port_label('output',4, 'MCU_DC_Link_Current'); port_label('output',5, 'Status');
  CanRx3 : S-Function  FunctionName=NsiCan_Rx_Ext  Parameters=data_can,channel,msg_name,ident,ident_type,dlc,signals,is_trigger,is_physical,is_canfd,is_rxgw  SFunctionDeploymentMode=off  EnableBusSupport=off  mask(MUXlink Can Rx){data_can=1;HIGH_SPEED;500Kbps;120 Ohm;C:\Users\TBRe-admin\Documents\MATLAB\TBRe18_DBC_190304.dbc;0;;;1;LOW_SPEED;125Kbps;560 Ohm;C:\Users\TBRe-admin\Documents\MATLAB\TBRe18_DBC_190304.dbc;0;;;0;HIGH_SPEED;1000Kbps;120 Ohm;D:\TOOLS\MUXLINK\R2011b\MUXlink\misc\BASE_CAN_MUXLAB4.dbc;0;;;0;HIGH_SPEED;500Kbps;120 Ohm;D:\TOOLS\MUXLINK\R2011b\MUXlink\misc\j1939_adapt.dbc;0;;;0;HIGH_SPEED;1000Kbps;No;D:\TOOLS\MUXLINK\R2011b\MUXlink\misc\BASE_CAN_MUXLAB4.dbc;0;;, channel=1, msg_name=MCU_TPDO1, ident=0x181, ident_type=STD, dlc=8, signals=MCU_Torque_Actual_Value;1;40;-16;1.000000;0.000000;_, is_trigger=0, is_physical=0, is_canfd=0, is_rxgw=0}
      mask prompts: data_can "data can"; msg_name "msg name"
      mask help: Receive a frame from a CAN channel.
      mask init:
      | NsiCan_Rx_Ext_InitializationFcn();
      settings: OpenFcn=NsiCan_Rx_Ext_OpenFcn();
      mask Help:
      | eval('block=get_param(gcb, ''RTWdata'');')
      | web([docroot '\toolbox\MUXlink\html\blocks/' block.MUXlink_BlockType '.html'])
      mask Callback data_can: NsiCan_Rx_Ext_ApplyFcn(1);
      mask Callback channel: NsiCan_Rx_Ext_ApplyFcn(2);
      mask Callback msg_name: NsiCan_Rx_Ext_ApplyFcn(3);
      mask Callback ident: NsiCan_Rx_Ext_ApplyFcn(4);
      mask Callback ident_type: NsiCan_Rx_Ext_ApplyFcn(5);
      mask Callback dlc: NsiCan_Rx_Ext_ApplyFcn(6);
      mask Callback signals: NsiCan_Rx_Ext_ApplyFcn(7);
      mask Callback is_trigger: NsiCan_Rx_Ext_ApplyFcn(8);
      mask Callback is_physical: NsiCan_Rx_Ext_ApplyFcn(9);
      mask Callback is_canfd: NsiCan_Rx_Ext_ApplyFcn(10);
      mask Callback is_rxgw: NsiCan_Rx_Ext_ApplyFcn(11);
      mask Display: image(imread('nsi.bmp'));text(0.5, 0.3, 'RX_MCU_TPDO1_CAN1', 'horizontalAlignment', 'center', 'verticalAlignment', 'base');plot([0.05 0.05 0.05 0.05 0.05 0.05 0.05 0.05 0.05 0.05]); port_label('output',1, 'MCU_Torque_Actual_Value'); port_label('output',2, 'Status');
  CanRx4 : S-Function  FunctionName=NsiCan_Rx_Ext  Parameters=data_can,channel,msg_name,ident,ident_type,dlc,signals,is_trigger,is_physical,is_canfd,is_rxgw  SFunctionDeploymentMode=off  EnableBusSupport=off  mask(MUXlink Can Rx){data_can=1;HIGH_SPEED;500Kbps;120 Ohm;X:\MechEng\Final Year Projects\TBRe\TBRe-19\3. Technical\3.04 LV Systems\05 ECU\TBRe18_DBC_190304.dbc;0;;;1;LOW_SPEED;125Kbps;560 Ohm;X:\MechEng\Final Year Projects\TBRe\TBRe-19\3. Technical\3.04 LV Systems\05 ECU\TBRe18_DBC_190304.dbc;0;;;0;HIGH_SPEED;1000Kbps;120 Ohm;D:\TOOLS\MUXLINK\R2011b\MUXlink\misc\BASE_CAN_MUXLAB4.dbc;0;;;0;HIGH_SPEED;500Kbps;120 Ohm;D:\TOOLS\MUXLINK\R2011b\MUXlink\misc\j1939_adapt.dbc;0;;;0;HIGH_SPEED;1000Kbps;No;D:\TOOLS\MUXLINK\R2011b\MUXlink\misc\BASE_CAN_MUXLAB4.dbc;0;;, channel=1, msg_name=MCU_SDO_Response, ident=0x581, ident_type=STD, dlc=8, signals=SDO_Specifier;1;0;8;1.000000;0.000000;_;MCU_OD_Sub_Index;1;24;8;1.000000;0.000000;_;MCU_OD_Index;1;8;16;1.000000;0.000000;_;SDO_Data;1;32;32;1.000000;0.000000;_, is_trigger=0, is_physical=0, is_canfd=0, is_rxgw=0}
      mask prompts: data_can "data can"; msg_name "msg name"
      mask help: Receive a frame from a CAN channel.
      mask init:
      | NsiCan_Rx_Ext_InitializationFcn();
      settings: OpenFcn=NsiCan_Rx_Ext_OpenFcn();
      mask Help:
      | eval('block=get_param(gcb, ''RTWdata'');')
      | web([docroot '\toolbox\MUXlink\html\blocks/' block.MUXlink_BlockType '.html'])
      mask Callback data_can: NsiCan_Rx_Ext_ApplyFcn(1);
      mask Callback channel: NsiCan_Rx_Ext_ApplyFcn(2);
      mask Callback msg_name: NsiCan_Rx_Ext_ApplyFcn(3);
      mask Callback ident: NsiCan_Rx_Ext_ApplyFcn(4);
      mask Callback ident_type: NsiCan_Rx_Ext_ApplyFcn(5);
      mask Callback dlc: NsiCan_Rx_Ext_ApplyFcn(6);
      mask Callback signals: NsiCan_Rx_Ext_ApplyFcn(7);
      mask Callback is_trigger: NsiCan_Rx_Ext_ApplyFcn(8);
      mask Callback is_physical: NsiCan_Rx_Ext_ApplyFcn(9);
      mask Callback is_canfd: NsiCan_Rx_Ext_ApplyFcn(10);
      mask Callback is_rxgw: NsiCan_Rx_Ext_ApplyFcn(11);
      mask Display: image(imread('nsi.bmp'));text(0.5, 0.3, 'RX_MCU_SDO_Response_CAN1', 'horizontalAlignment', 'center', 'verticalAlignment', 'base');plot([0.05 0.05 0.05 0.05 0.05 0.05 0.05 0.05 0.05 0.05]); port_label('output',1, 'SDO_Specifier'); port_label('output',2, 'MCU_OD_Sub_Index'); port_label('output',3, 'MCU_OD_Index'); port_label('output',4, 'SDO_Data'); port_label('output',5, 'Status');
  Init : Subsystem  mask(System Initialize){}
      mask help: Add code to a systems Initialize function
      settings: CopyFcn=cccopyfcn(gcb)  OpenFcn=ccopenfcn('System Initialize Function')
      mask Help: This block contains text fields to insert custom user code sections at the declaration, execution and exit sections of the systems initialize function.  By placing this block inside a subsytem, the custom user code will appear in that subsystems function.
      mask Display: disp('I()')
  Task : S-Function  FunctionName=NsiSys_TaskREF  Parameters=task_initialised,task_periodic, task_sampletime,task_name,task_event,task_offset  SFunctionDeploymentMode=off  EnableBusSupport=off  mask(task definition){task_initialised=on, task_periodic=on, task_sampletime=[0.05], task_offset=0, task_name=High_Priority_CAN_RX, task_event=on}
      mask prompts: task_initialised "task initialised"; task_periodic "Is Periodic"; task_sampletime "Task sample time"; task_offset "Task Offset"; task_name "Task name"; task_event "Is event"
      mask help:
      | Permit to provide all parameters associated to a MUXLINK task.
      | Task can be executed periodicaly and/or on event detection.
      | If task is periodic:
      | Task sample time specify the execution period in mS [0.001   6000]
      | Task Offset specify the offset applied to the execution period
      | Task Offset < Task sample time
      mask init:
      | NsiSys_TaskREF_InitializationFcn();
      settings: OpenFcn=NsiSys_Task_OpenFcn();
      mask Callback task_initialised: NsiSys_TaskREF_ApplyFcn(1);
      mask Callback task_periodic: NsiSys_TaskREF_ApplyFcn(2);
      mask Callback task_sampletime: NsiSys_TaskREF_ApplyFcn(3);
      mask Callback task_offset: NsiSys_TaskREF_ApplyFcn(6);
      mask Callback task_name: NsiSys_TaskREF_ApplyFcn(4);
      mask Callback task_event: NsiSys_TaskREF_ApplyFcn(5);
      mask Display: text(0.5, 0.8, 't()', 'horizontalAlignment', 'center', 'verticalAlignment', 'base');text(0.5, 0.2, '/ 50.0ms / 0.0ms /', 'horizontalAlignment', 'center', 'verticalAlignment', 'base');text(0.5, 0.4, 'Event', 'horizontalAlignment', 'center', 'verticalAlignment', 'base');
  Terminator : Terminator
  Terminator1 : Terminator
  Terminator2 : Terminator
  Out1 : Outport
  wires:
  Bus Creator1/1 -> Out1/1  "HAL_MCU"
  CanRx2/4 -> Bus Creator1/9  "MCU_DC_Link_Current"
  CanRx2/5 -> Terminator1/1
  CanRx3/2 -> Terminator/1
  CanRx4/4 -> Bus Creator1/5  "SDO_Data"
  CanRx4/5 -> Terminator2/1
  CanRx4/1 -> Bus Creator1/2  "SDO_Response_Command"
  CanRx4/2 -> Bus Creator1/3  "OD_Sub_Index"
  CanRx2/3 -> Bus Creator1/8  "MCU_DC_Link_Voltage"
  CanRx3/1 -> Bus Creator1/1  "MCU_Target_Torque"
  CanRx4/3 -> Bus Creator1/4  "OD_Index"
  CanRx2/2 -> Bus Creator1/7  "MCU_Temp"
  CanRx2/1 -> Bus Creator1/6  "Motor_Temp"

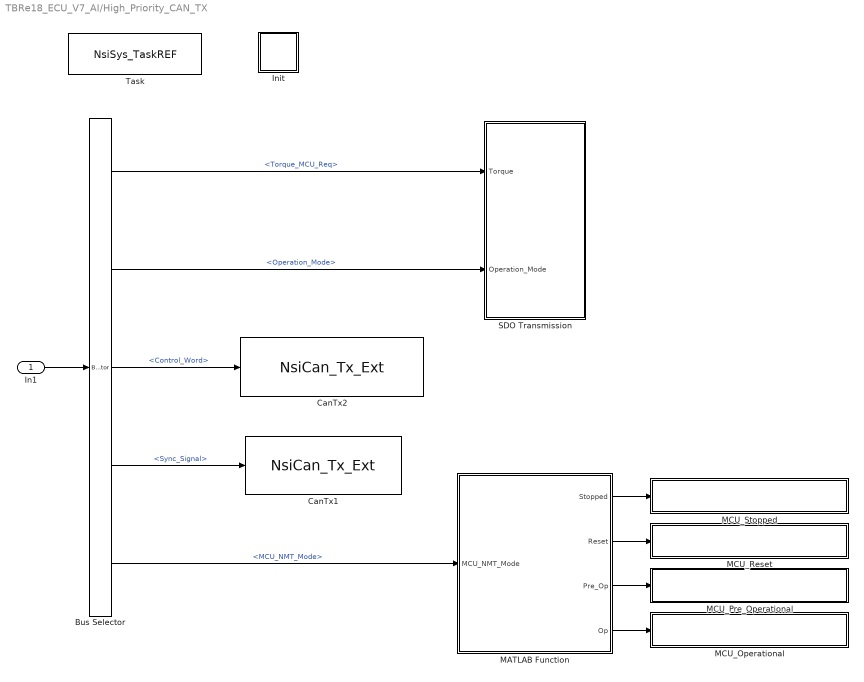
== system TBRe18_ECU_V7_AI/High_Priority_CAN_TX ==
  In1 : Inport
  Bus Selector : BusSelector  OutputSignals=Drive_Data.Torque_MCU_Req,Vehicle_Operation_Data.Operation_Mode,Drive_Data.Control_Word,Drive_Data.Sync_Signal,Vehicle_Operation_Data.MCU_NMT_Mode
  CanTx1 : S-Function  FunctionName=NsiCan_Tx_Ext  Parameters=data_can,channel,msg_name,ident,ident_type,dlc,signals,is_physical,is_canfd,is_crc  SFunctionDeploymentMode=off  EnableBusSupport=off  mask(MUXlink Can Tx){data_can=1;HIGH_SPEED;500Kbps;120 Ohm;C:\Users\TBRe-admin\Documents\MATLAB\TBRe18_DBC_190304.dbc;0;;;1;LOW_SPEED;125Kbps;560 Ohm;C:\Users\TBRe-admin\Documents\MATLAB\TBRe18_DBC_190304.dbc;0;;;0;HIGH_SPEED;1000Kbps;120 Ohm;D:\TOOLS\MUXLINK\R2011b\MUXlink\misc\BASE_CAN_MUXLAB4.dbc;0;;;0;HIGH_SPEED;500Kbps;120 Ohm;D:\TOOLS\MUXLINK\R2011b\MUXlink\misc\j1939_adapt.dbc;0;;;0;HIGH_SPEED;1000Kbps;No;D:\TOOLS\MUXLINK\R2011b\MUXlink\misc\BASE_CAN_MUXLAB4.dbc;0;;, channel=1, msg_name=MCU_Sync_MSG, ident=0x080, ident_type=STD, dlc=1, signals=Sync_Command;1;0;8;1.000000;0.000000;_, is_physical=0, is_canfd=0, is_crc=0}
      mask prompts: data_can "data can"; msg_name "msg name"
      mask help: Transmit a frame on a CAN Channel.
      mask init:
      | NsiCan_Tx_Ext_InitializationFcn();
      settings: OpenFcn=NsiCan_Tx_Ext_OpenFcn();
      mask Help:
      | eval('block=get_param(gcb, ''RTWdata'');')
      | web([docroot '\toolbox\MUXlink\html\blocks/' block.MUXlink_BlockType '.html'])
      mask Callback data_can: NsiCan_Tx_Ext_ApplyFcn(1);
      mask Callback channel: NsiCan_Tx_Ext_ApplyFcn(2);
      mask Callback msg_name: NsiCan_Tx_Ext_ApplyFcn(3);
      mask Callback ident: NsiCan_Tx_Ext_ApplyFcn(4);
      mask Callback ident_type: NsiCan_Tx_Ext_ApplyFcn(5);
      mask Callback dlc: NsiCan_Tx_Ext_ApplyFcn(6);
      mask Callback signals: NsiCan_Tx_Ext_ApplyFcn(7);
      mask Callback is_physical: NsiCan_Tx_Ext_ApplyFcn(7);
      mask Callback is_canfd: NsiCan_Tx_Ext_ApplyFcn(7);
      mask Callback is_crc: NsiCan_Tx_Ext_ApplyFcn(7);
      mask Display: image(imread('nsi.bmp'));text(0.5, 0.1, 'TX_MCU_Sync_MSG_CAN1', 'horizontalAlignment', 'center', 'verticalAlignment', 'base');plot([0.05 0.05 0.05 0.05 0.05 0.05 0.05 0.05 0.05 0.05]); port_label('input',1, 'Sync_Command');
  CanTx2 : S-Function  FunctionName=NsiCan_Tx_Ext  Parameters=data_can,channel,msg_name,ident,ident_type,dlc,signals,is_physical,is_canfd,is_crc  SFunctionDeploymentMode=off  EnableBusSupport=off  mask(MUXlink Can Tx){data_can=1;HIGH_SPEED;500Kbps;120 Ohm;C:\Users\TBRe-admin\Documents\MATLAB\TBRe18_DBC_190304.dbc;0;;;1;LOW_SPEED;125Kbps;560 Ohm;C:\Users\TBRe-admin\Documents\MATLAB\TBRe18_DBC_190304.dbc;0;;;0;HIGH_SPEED;1000Kbps;120 Ohm;D:\TOOLS\MUXLINK\R2011b\MUXlink\misc\BASE_CAN_MUXLAB4.dbc;0;;;0;HIGH_SPEED;500Kbps;120 Ohm;D:\TOOLS\MUXLINK\R2011b\MUXlink\misc\j1939_adapt.dbc;0;;;0;HIGH_SPEED;1000Kbps;No;D:\TOOLS\MUXLINK\R2011b\MUXlink\misc\BASE_CAN_MUXLAB4.dbc;0;;, channel=1, msg_name=MCU_RPDO1, ident=0x201, ident_type=STD, dlc=8, signals=MCU_ControlWord;1;0;16;1.000000;0.000000;_, is_physical=0, is_canfd=0, is_crc=0}
      mask prompts: data_can "data can"; msg_name "msg name"
      mask help: Transmit a frame on a CAN Channel.
      mask init:
      | NsiCan_Tx_Ext_InitializationFcn();
      settings: OpenFcn=NsiCan_Tx_Ext_OpenFcn();
      mask Help:
      | eval('block=get_param(gcb, ''RTWdata'');')
      | web([docroot '\toolbox\MUXlink\html\blocks/' block.MUXlink_BlockType '.html'])
      mask Callback data_can: NsiCan_Tx_Ext_ApplyFcn(1);
      mask Callback channel: NsiCan_Tx_Ext_ApplyFcn(2);
      mask Callback msg_name: NsiCan_Tx_Ext_ApplyFcn(3);
      mask Callback ident: NsiCan_Tx_Ext_ApplyFcn(4);
      mask Callback ident_type: NsiCan_Tx_Ext_ApplyFcn(5);
      mask Callback dlc: NsiCan_Tx_Ext_ApplyFcn(6);
      mask Callback signals: NsiCan_Tx_Ext_ApplyFcn(7);
      mask Callback is_physical: NsiCan_Tx_Ext_ApplyFcn(7);
      mask Callback is_canfd: NsiCan_Tx_Ext_ApplyFcn(7);
      mask Callback is_crc: NsiCan_Tx_Ext_ApplyFcn(7);
      mask Display: image(imread('nsi.bmp'));text(0.5, 0.1, 'TX_MCU_RPDO1_CAN1', 'horizontalAlignment', 'center', 'verticalAlignment', 'base');plot([0.05 0.05 0.05 0.05 0.05 0.05 0.05 0.05 0.05 0.05]); port_label('input',1, 'MCU_ControlWord');
  Init : Subsystem  mask(System Initialize){}
      mask help: Add code to a systems Initialize function
      settings: CopyFcn=cccopyfcn(gcb)  OpenFcn=ccopenfcn('System Initialize Function')
      mask Help: This block contains text fields to insert custom user code sections at the declaration, execution and exit sections of the systems initialize function.  By placing this block inside a subsytem, the custom user code will appear in that subsystems function.
      mask Display: disp('I()')
  MATLAB Function : MATLAB Function  TreatAsAtomicUnit=on
  MCU_Operational : Subsystem
  MCU_Pre_Operational : Subsystem
  MCU_Reset : Subsystem
  MCU_Stopped : Subsystem
  SDO Transmission : Subsystem
  Task : S-Function  FunctionName=NsiSys_TaskREF  Parameters=task_initialised,task_periodic, task_sampletime,task_name,task_event,task_offset  SFunctionDeploymentMode=off  EnableBusSupport=off  mask(task definition){task_initialised=on, task_periodic=on, task_sampletime=[0.05], task_offset=0.02, task_name=High_Priority_CAN_TX, task_event=on}
      mask prompts: task_initialised "task initialised"; task_periodic "Is Periodic"; task_sampletime "Task sample time"; task_offset "Task Offset"; task_name "Task name"; task_event "Is event"
      mask help:
      | Permit to provide all parameters associated to a MUXLINK task.
      | Task can be executed periodicaly and/or on event detection.
      | If task is periodic:
      | Task sample time specify the execution period in mS [0.001   6000]
      | Task Offset specify the offset applied to the execution period
      | Task Offset < Task sample time
      mask init:
      | NsiSys_TaskREF_InitializationFcn();
      settings: OpenFcn=NsiSys_Task_OpenFcn();
      mask Callback task_initialised: NsiSys_TaskREF_ApplyFcn(1);
      mask Callback task_periodic: NsiSys_TaskREF_ApplyFcn(2);
      mask Callback task_sampletime: NsiSys_TaskREF_ApplyFcn(3);
      mask Callback task_offset: NsiSys_TaskREF_ApplyFcn(6);
      mask Callback task_name: NsiSys_TaskREF_ApplyFcn(4);
      mask Callback task_event: NsiSys_TaskREF_ApplyFcn(5);
      mask Display: text(0.5, 0.8, 't()', 'horizontalAlignment', 'center', 'verticalAlignment', 'base');text(0.5, 0.2, '/ 50.0ms / 20.0ms /', 'horizontalAlignment', 'center', 'verticalAlignment', 'base');text(0.5, 0.4, 'Event', 'horizontalAlignment', 'center', 'verticalAlignment', 'base');
  wires:
  MATLAB Function/2(Reset) -> MCU_Reset/Trigger
  Bus Selector/5 -> MATLAB Function/1(MCU_NMT_Mode)  "<MCU_NMT_Mode>"
  Bus Selector/1 -> SDO Transmission/1(Torque)  "<Torque_MCU_Req>"
  Bus Selector/4 -> CanTx1/1  "<Sync_Signal>"
  MATLAB Function/1(Stopped) -> MCU_Stopped/Trigger
  MATLAB Function/4(Op) -> MCU_Operational/Trigger
  In1/1 -> Bus Selector/1
  Bus Selector/3 -> CanTx2/1  "<Control_Word>"
  MATLAB Function/3(Pre_Op) -> MCU_Pre_Operational/Trigger
  Bus Selector/2 -> SDO Transmission/2(Operation_Mode)  "<Operation_Mode>"
